simulink subsystem "rss_ShOffFlgConfSens"  (R2023a)
settings: Solver=VariableStepAuto  StartTime=0.0  StopTime=10.0  RelTol=1e-3
undefined symbols (not defined in the file): ENM_SYS_STATUS
libraries: simulink x4
settings Model: Creator=xiaoqiang.yuan  LastModifiedBy=xiaoqiang.yuan

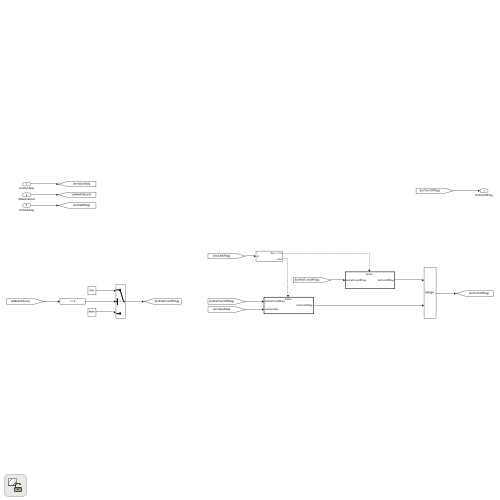
[thumbnail: Simulink's stored preview of the top-level diagram]
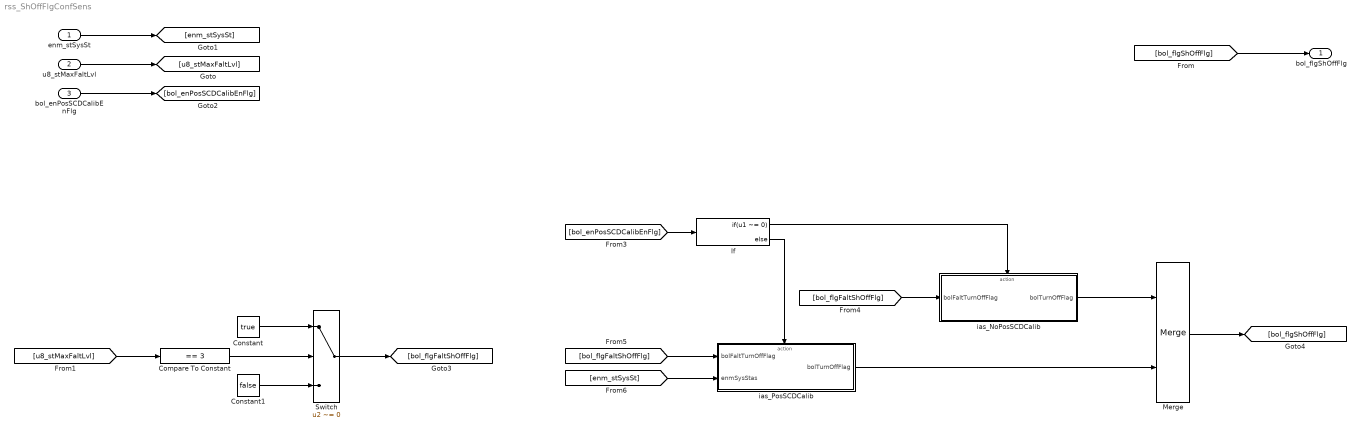
== system rss_ShOffFlgConfSens ==
  enm_stSysSt : Inport  OutDataTypeStr=Enum: ENM_SYS_STATUS
  u8_stMaxFaltLvl : Inport  Port=2  OutDataTypeStr=uint8
  bol_enPosSCDCalibEnFlg : Inport  Port=3  OutDataTypeStr=boolean
  Compare To Constant : simulink/Logic and Bit Operations/Compare To Constant  relop===  const=3  OutDataTypeStr=boolean
  Constant : Constant  Value=true  OutDataTypeStr=boolean
  Constant1 : Constant  Value=false  OutDataTypeStr=boolean
  If : If  IfExpression=u1 ~= 0
  Merge : Merge
  Switch : Switch  Criteria=u2 ~= 0  SaturateOnIntegerOverflow=off  InputSameDT=off
  ias_NoPosSCDCalib : Subsystem  TreatAsAtomicUnit=on
  ias_PosSCDCalib : Subsystem  TreatAsAtomicUnit=on
  bol_flgShOffFlg : Outport  OutDataTypeStr=boolean
  wires:
  enm_stSysSt/1 -> [enm_stSysSt]
  bol_enPosSCDCalibEnFlg/1 -> [bol_enPosSCDCalibEnFlg]
  [bol_flgShOffFlg] -> bol_flgShOffFlg/1
  [bol_enPosSCDCalibEnFlg] -> If/1
  If/1 -> ias_NoPosSCDCalib/Action
  [bol_flgFaltShOffFlg] -> ias_NoPosSCDCalib/1(bolFaltTurnOffFlag)
  ias_NoPosSCDCalib/1(bolTurnOffFlag) -> Merge/1
  Merge/1 -> [bol_flgShOffFlg]
  If/2 -> ias_PosSCDCalib/Action
  [bol_flgFaltShOffFlg] -> ias_PosSCDCalib/1(bolFaltTurnOffFlag)
  [enm_stSysSt] -> ias_PosSCDCalib/2(enmSysStas)
  ias_PosSCDCalib/1(bolTurnOffFlag) -> Merge/2
  [u8_stMaxFaltLvl] -> Compare To Constant/1
  Compare To Constant/1 -> Switch/2
  Constant1/1 -> Switch/3
  Constant/1 -> Switch/1
  Switch/1 -> [bol_flgFaltShOffFlg]
  u8_stMaxFaltLvl/1 -> [u8_stMaxFaltLvl]

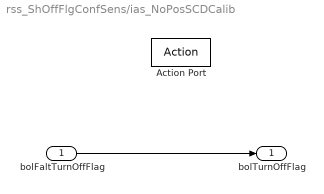
== system rss_ShOffFlgConfSens/ias_NoPosSCDCalib ==
  bolFaltTurnOffFlag : Inport
  Action Port : ActionPort
  bolTurnOffFlag : Outport
  wires:
  bolFaltTurnOffFlag/1 -> bolTurnOffFlag/1

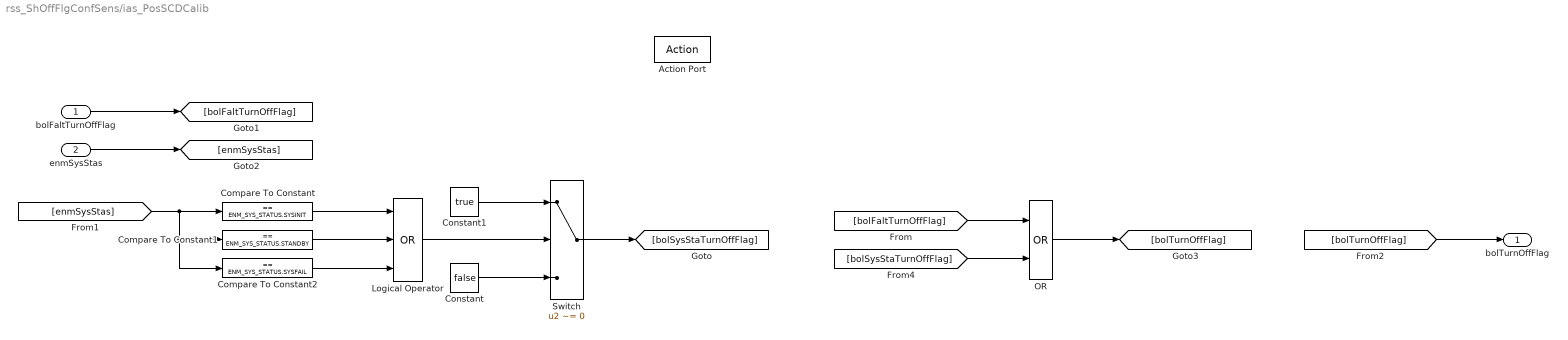
== system rss_ShOffFlgConfSens/ias_PosSCDCalib ==
  bolFaltTurnOffFlag : Inport
  enmSysStas : Inport  Port=2
  Action Port : ActionPort
  Compare To Constant : simulink/Logic and Bit Operations/Compare To Constant  relop===  const=ENM_SYS_STATUS.SYSINIT  OutDataTypeStr=boolean
  Compare To Constant1 : simulink/Logic and Bit Operations/Compare To Constant  relop===  const=ENM_SYS_STATUS.STANDBY  OutDataTypeStr=boolean
  Compare To Constant2 : simulink/Logic and Bit Operations/Compare To Constant  relop===  const=ENM_SYS_STATUS.SYSFAIL  OutDataTypeStr=boolean
  Constant : Constant  Value=false  OutDataTypeStr=boolean
  Constant1 : Constant  Value=true  OutDataTypeStr=boolean
  Logical Operator : Logic  Operator=OR  Inputs=3  AllPortsSameDT=off  OutDataTypeStr=boolean
  OR : Logic  Operator=OR  AllPortsSameDT=off  OutDataTypeStr=boolean
  Switch : Switch  Criteria=u2 ~= 0  SaturateOnIntegerOverflow=off  InputSameDT=off
  bolTurnOffFlag : Outport
  wires:
  Compare To Constant2/1 -> Logical Operator/3
  Constant1/1 -> Switch/1
  Constant/1 -> Switch/3
  [bolTurnOffFlag] -> bolTurnOffFlag/1
  OR/1 -> [bolTurnOffFlag]
  [bolFaltTurnOffFlag] -> OR/1
  enmSysStas/1 -> [enmSysStas]
  bolFaltTurnOffFlag/1 -> [bolFaltTurnOffFlag]
  [bolSysStaTurnOffFlag] -> OR/2
  Switch/1 -> [bolSysStaTurnOffFlag]
  Logical Operator/1 -> Switch/2
  [enmSysStas] -> Compare To Constant/1, Compare To Constant1/1, Compare To Constant2/1
  Compare To Constant1/1 -> Logical Operator/2
  Compare To Constant/1 -> Logical Operator/1
